simulink model "example_model"  (R2017b)
settings: Solver=VariableStepAuto  StartTime=0.0  StopTime=10.0  RelTol=1e-3
settings Model: Creator=vanch  LastModifiedBy=vanch

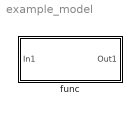
== system example_model ==
  func : Subsystem

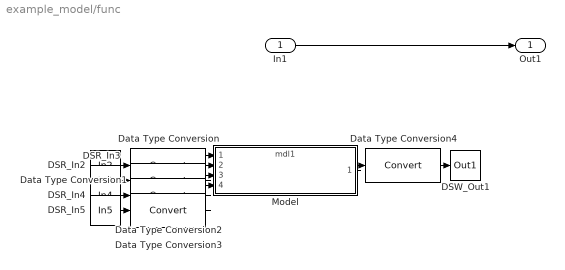
== system example_model/func ==
  In1 : Inport
  DSR_In2 : DataStoreRead  DataStoreName=In2
  DSR_In3 : DataStoreRead  DataStoreName=In3
  DSR_In4 : DataStoreRead  DataStoreName=In4
  DSR_In5 : DataStoreRead  DataStoreName=In5
  DSW_Out1 : DataStoreWrite  DataStoreName=Out1
  Data Type Conversion{,1..4} (5 alike) : DataTypeConversion
  Model : ModelReference  ModelNameDialog=mdl1  SimulationMode=Normal  ModelReferenceVersion=1.1
  Out1 : Outport
  wires:
  In1/1 -> Out1/1
  Data Type Conversion/1 -> Model/1
  DSR_In2/1 -> Data Type Conversion/1
  Data Type Conversion1/1 -> Model/2
  DSR_In3/1 -> Data Type Conversion1/1
  Data Type Conversion2/1 -> Model/3
  DSR_In4/1 -> Data Type Conversion2/1
  Data Type Conversion3/1 -> Model/4
  DSR_In5/1 -> Data Type Conversion3/1
  Model/1 -> Data Type Conversion4/1
  Data Type Conversion4/1 -> DSW_Out1/1
